simulink model "segway_system"  (R2020a)
settings: Solver=FixedStepAuto  StartTime=0.0  StopTime=inf  FixedStep=.03  RelTol=1e-3
values from neighbouring files (symbols this model uses):
  K_lqr = lqr(A,B,Q,R)    [segway_m.m]
  Rw = .0216    (= 0.0216)    [segode.m]    (also in segode2.m; segway_m.m)
undefined symbols (not defined in the file or in its folder): DiscIntNeverNeededParam
libraries: MinSegLibrary_M1V4 x2, simulink x1
settings Model: SILPILModeSetting=veronly  ExtModeTrigDuration=2  Creator=super  LastModifiedBy=super
settings DataIOCC: SaveFormat=Array  ReturnWorkspaceOutputs=off
settings OptimizationCC: EnhancedBackFolding=on  PassReuseOutputArgsAs=Individual arguments  ZeroExternalMemoryAtStartup=off  ZeroInternalMemoryAtStartup=off  MaxStackSize=64  OptimizeBlockOrder=speed  DifferentSizesBufferReuse=on  OptimizationCustomize=off  EfficientTunableParamExpr=on
settings DebuggingCC: ParameterTunabilityLossMsg=error
settings HardwareCC: ProdBitPerInt=16  ProdBitPerPointer=16  ProdBitPerSizeT=16  ProdBitPerPtrDiffT=16  ProdLargestAtomicFloat=None  ProdWordSize=8  ProdHWDeviceType=Atmel->AVR  UseEmbeddedCoderFeatures=off  UseSimulinkCoderFeatures=off
settings SFSimCC: MATLABDynamicMemAlloc=off
settings RTWCC: SystemTargetFile=ert.tlc  HardwareBoard=Arduino Mega 2560  TLCOptions=-aInlineSetEventsForThisBaseRateFcn=TLC_FALSE -aSuppressMultiTaskScheduler=TLC_FALSE -aRateBasedStepFcn=1  TemplateMakefile=ert_default_tmf  Toolchain=Arduino AVR
settings CodeAppCC: ForceParamTrailComments=on  IgnoreCustomStorageClasses=off  OperatorAnnotations=on  SimulinkDataObjDesc=on  SFDataObjDesc=on  InsertBlockDesc=on
settings ERTTargetCC: SupportContinuousTime=on  SupportNonInlinedSFcns=on  SupportVariableSizeSignals=on  ExtModeStaticAllocSize=2048

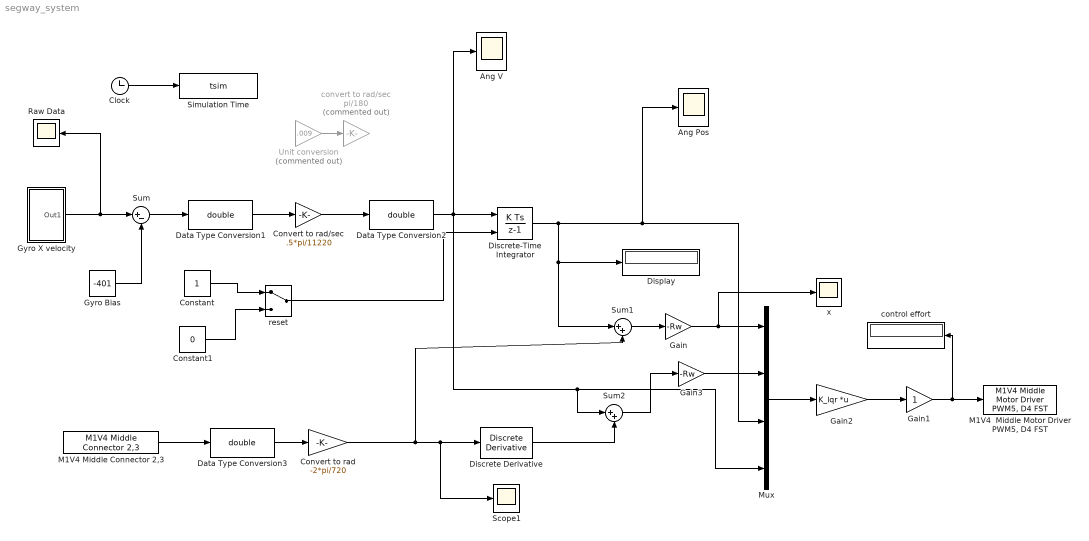
== system segway_system ==
  Ang Pos : Scope
  Ang V : Scope
  Clock : Clock
  Constant : Constant
  Constant1 : Constant  Value=0
  Convert to rad : Gain  Gain=-2*pi/720
  Convert to rad/sec : Gain  Gain=.5*pi/11220
  Data Type Conversion1 : DataTypeConversion  OutDataTypeStr=double
  Data Type Conversion2 : DataTypeConversion  OutDataTypeStr=double
  Data Type Conversion3 : DataTypeConversion  OutDataTypeStr=double
  Discrete Derivative : simulink/Discrete/Discrete Derivative  gainval=1.0  ICPrevScaledInput=0.0  OutMin=[]  OutMax=[]  OutDataType=fixdt(1, 16)  OutScaling=2^-10  DoSatur=off
  Discrete-Time Integrator : DiscreteIntegrator  ExternalReset=either  SampleTime=-1  ICPrevOutput=DiscIntNeverNeededParam  ICPrevScaledInput=DiscIntNeverNeededParam
  Display : Display
  Gain : Gain  Gain=-Rw
  Gain1 : Gain
  Gain2 : Gain  Gain=K_lqr  Multiplication=Matrix(K*u)
  Gain3 : Gain  Gain=-Rw
  Gyro Bias : Constant  Value=-401
  Gyro X velocity : Subsystem
  "M1V4  Middle Motor Driver PWM5, D4 FST" : MinSegLibrary_M1V4/M1V4  Middle Motor Driver PWM5, D4 FST  Vsupply=3.9
      settings: SourceProductName=Rensselaer Arduino Support Package
  M1V4 Middle Connector 2,3 : MinSegLibrary_M1V4/M1V4 Middle Connector 2,3  Encoder=0  PinA=3  PinB=2
      settings: SourceProductName=Rensselaer Arduino Support Package
  Mux : Mux
  Raw Data : Scope
  Scope1 : Scope
  Simulation Time : ToWorkspace  VariableName=tsim  SampleTime=-1
  Sum : Sum  Inputs=|+-
  Sum1 : Sum  Inputs=|++
  Sum2 : Sum  Inputs=|++
  Unit conversion : Gain  Commented=on  Gain=.009
  control effort : Display
  convert to rad/sec : Gain  Commented=on  Gain=pi/180
  reset : ManualSwitch
  x : Scope
  wires:
  Clock/1 -> Simulation Time/1
  Sum/1 -> Data Type Conversion1/1
  Constant1/1 -> reset/2
  Gyro X velocity/1(Out1) -> Raw Data/1, Sum/1
  Constant/1 -> reset/1
  Gyro Bias/1 -> Sum/2
  reset/1 -> Discrete-Time Integrator/2
  Discrete-Time Integrator/1 -> Display/1, Sum1/1, Mux/3, Ang Pos/1
  Discrete Derivative/1 -> Sum2/2
  Gain3/1 -> Mux/2
  Unit conversion/1 -> convert to rad/sec/1
  Mux/1 -> Gain2/1
  Data Type Conversion2/1 -> Ang V/1, Sum2/1, Mux/4, Discrete-Time Integrator/1
  Gain1/1 -> control effort/1, "M1V4  Middle Motor Driver PWM5, D4 FST"/1
  Sum1/1 -> Gain/1
  Gain/1 -> x/1, Mux/1
  Sum2/1 -> Gain3/1
  Gain2/1 -> Gain1/1
  Data Type Conversion1/1 -> Convert to rad/sec/1
  Convert to rad/sec/1 -> Data Type Conversion2/1
  Data Type Conversion3/1 -> Convert to rad/1
  M1V4 Middle Connector 2,3/1 -> Data Type Conversion3/1
  Convert to rad/1 -> Sum1/2, Scope1/1, Discrete Derivative/1

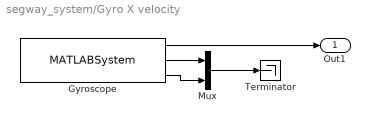
== system segway_system/Gyro X velocity ==
  Gyroscope : MATLABSystem  System=soMPU6050Gyro  DLPFmode=5
      mask Type: soMPU6050Gyro
      mask Display:
      | disp('soMPU6050Gyro');
      | port_label('output',1,'xvel');
      | port_label('output',2,'yvel');
      | port_label('output',3,'zvel');
  Mux : Mux  Inputs=2
  Terminator : Terminator
  Out1 : Outport
  wires:
  Mux/1 -> Terminator/1
  Gyroscope/3 -> Mux/2
  Gyroscope/2 -> Mux/1
  Gyroscope/1 -> Out1/1
